simulink model "Simulation_CircularSensor"  (R2020a)
settings: Solver=VariableStepAuto  StartTime=0.0  StopTime=10  RelTol=1e-3
values from neighbouring files (symbols this model uses):
  L = 0    [CircularSensorTest.m]    (also in init.m = 0 * scale; polyTest.m = 10)
  Pixels = [0 0 0 0 0 0 0 0 0 0 0 0 ... (1000000 elements, 1000x1000)]    [CrossMap.mat]    (also in GenerateCourseData.m = zeros(Height, Width); Pixels.mat = [0 0 0 0 0 0 0 0 0 0 0 0 ... (19600 elements, 140x140)])
  scale = 1    [GenerateCourseData.m]
  SensorAngle = 60    [CircularSensorTest.m]    (also in init.m)
  SensorNumber = 3    [CircularSensorTest.m]    (also in animation2.m = evalin('base', 'SensorNumber'); init.m)
  SensorRadius = 40    [CircularSensorTest.m]    (also in init.m = 50 * scale)
  SensorRange = 20    [CircularSensorTest.m]    (also in animation2.m = evalin('base', 'SensorRange'); init.m = 25 * scale)
  Tvelo = 0.1    [init.m]
undefined symbols (not defined in the file or in its folder): DiscIntNeverNeededParam
settings Model: SimulationMode=rapid-accelerator  Creator=robot  LastModifiedBy=under

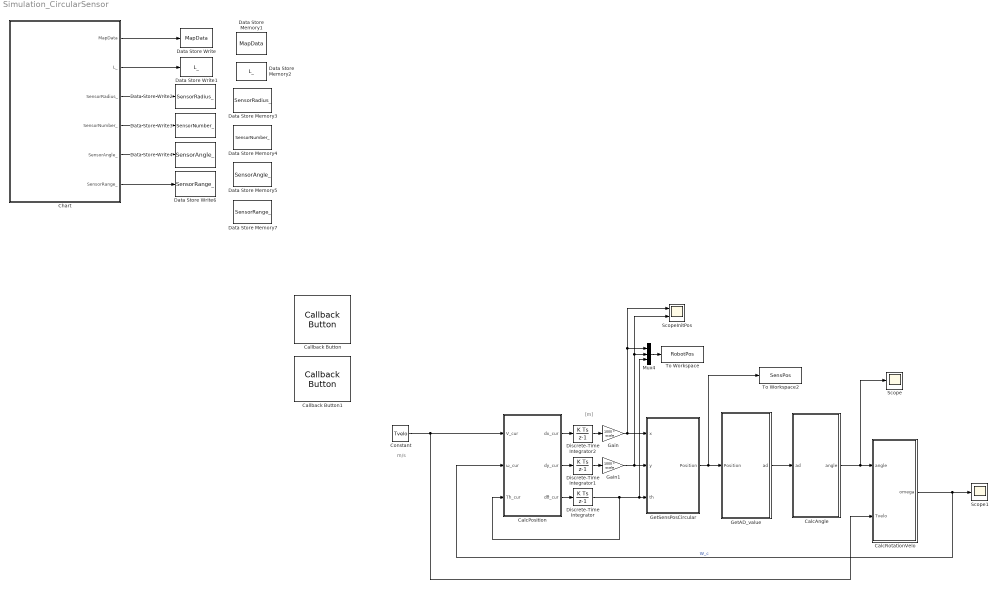
== system Simulation_CircularSensor ==
  note: [m]
  note: m/s
  CalcAngle : MATLAB Function  TreatAsAtomicUnit=on
  CalcPosition : Subsystem
  CalcRotationVelo : MATLAB Function  TreatAsAtomicUnit=on
  Callback Button : CallbackButton  ButtonText=Generata Course Data
      settings: ClickFcn=run('GenerateCourseData.m')
  Callback Button1 : CallbackButton  ButtonText=Initialize
      settings: ClickFcn=run('init.m')
  Chart : Stateflow chart  TreatAsAtomicUnit=on
  Constant : Constant  Value=Tvelo
  Data Store Memory1 : DataStoreMemory  DataStoreName=MapData  ReadBeforeWriteMsg=warning  WriteAfterWriteMsg=warning  WriteAfterReadMsg=warning  VectorParams1D=off  ShowAdditionalParam=off  OutDataTypeStr=double  Dimensions=[1000 ; 1000]
  Data Store Memory2 : DataStoreMemory  DataStoreName=L_  ReadBeforeWriteMsg=warning  WriteAfterWriteMsg=warning  WriteAfterReadMsg=warning  VectorParams1D=off  ShowAdditionalParam=off  OutDataTypeStr=double  Dimensions=1
  Data Store Memory3 : DataStoreMemory  DataStoreName=SensorRadius_  ReadBeforeWriteMsg=warning  WriteAfterWriteMsg=warning  WriteAfterReadMsg=warning  VectorParams1D=off  ShowAdditionalParam=off  OutDataTypeStr=double  Dimensions=1
  Data Store Memory4 : DataStoreMemory  DataStoreName=SensorNumber_  ReadBeforeWriteMsg=warning  WriteAfterWriteMsg=warning  WriteAfterReadMsg=warning  VectorParams1D=off  ShowAdditionalParam=off  OutDataTypeStr=double  Dimensions=1
  Data Store Memory5 : DataStoreMemory  DataStoreName=SensorAngle_  ReadBeforeWriteMsg=warning  WriteAfterWriteMsg=warning  WriteAfterReadMsg=warning  VectorParams1D=off  ShowAdditionalParam=off  OutDataTypeStr=double  Dimensions=1
  Data Store Memory7 : DataStoreMemory  DataStoreName=SensorRange_  ReadBeforeWriteMsg=warning  WriteAfterWriteMsg=warning  WriteAfterReadMsg=warning  VectorParams1D=off  ShowAdditionalParam=off  OutDataTypeStr=double  Dimensions=1
  Data Store Write : DataStoreWrite  DataStoreName=MapData
  Data Store Write1 : DataStoreWrite  DataStoreName=L_
  Data Store Write2 : DataStoreWrite  DataStoreName=SensorRadius_
  Data Store Write3 : DataStoreWrite  DataStoreName=SensorNumber_
  Data Store Write4 : DataStoreWrite  DataStoreName=SensorAngle_
  Data Store Write6 : DataStoreWrite  DataStoreName=SensorRange_
  Discrete-Time Integrator : DiscreteIntegrator  SampleTime=-1  ICPrevOutput=DiscIntNeverNeededParam  ICPrevScaledInput=DiscIntNeverNeededParam
  Discrete-Time Integrator1 : DiscreteIntegrator  InitialCondition=0.15  SampleTime=-1  ICPrevOutput=DiscIntNeverNeededParam  ICPrevScaledInput=DiscIntNeverNeededParam
  Discrete-Time Integrator2 : DiscreteIntegrator  InitialCondition=0.5  SampleTime=-1  ICPrevOutput=DiscIntNeverNeededParam  ICPrevScaledInput=DiscIntNeverNeededParam
  Gain : Gain  Gain=1000 * scale
  Gain1 : Gain  Gain=1000 * scale
  GetAD_value : MATLAB Function  TreatAsAtomicUnit=on
  GetSensPosCircular : MATLAB Function  TreatAsAtomicUnit=on
  Mux4 : Mux  Inputs=3
  Scope : Scope
  Scope1 : Scope
  ScopeInitPos : Scope  NumInputPorts=2
  To Workspace : ToWorkspace  VariableName=RobotPos  SampleTime=-1
  To Workspace2 : ToWorkspace  VariableName=SensPos  SaveFormat=Structure  SampleTime=-1
  wires:
  Constant/1 -> CalcPosition/1(V_cur), CalcRotationVelo/2(Tvelo)
  CalcPosition/3(dθ_cur) -> Discrete-Time Integrator/1
  Discrete-Time Integrator/1 -> CalcPosition/3(Th_cur), Mux4/3, GetSensPosCircular/3(th)
  Mux4/1 -> To Workspace/1
  GetSensPosCircular/1(Position) -> To Workspace2/1, GetAD_value/1(Position)
  Discrete-Time Integrator2/1 -> Gain/1
  Discrete-Time Integrator1/1 -> Gain1/1
  CalcPosition/1(dx_cur) -> Discrete-Time Integrator2/1
  CalcPosition/2(dy_cur) -> Discrete-Time Integrator1/1
  Gain/1 -> ScopeInitPos/1, Mux4/1, GetSensPosCircular/1(x)
  Gain1/1 -> ScopeInitPos/2, Mux4/2, GetSensPosCircular/2(y)
  Chart/1(MapData) -> Data Store Write/1
  Chart/2(L_) -> Data Store Write1/1
  Chart/3(SensorRadius_) -> Data Store Write2/1
  Chart/4(SensorNumber_) -> Data Store Write3/1
  Chart/5(SensorAngle_) -> Data Store Write4/1
  Chart/6(SensorRange_) -> Data Store Write6/1
  GetAD_value/1(ad) -> CalcAngle/1(ad)
  CalcAngle/1(angle) -> Scope/1, CalcRotationVelo/1(angle)
  CalcRotationVelo/1(omega) -> CalcPosition/2(ω_cur), Scope1/1  "W_c"

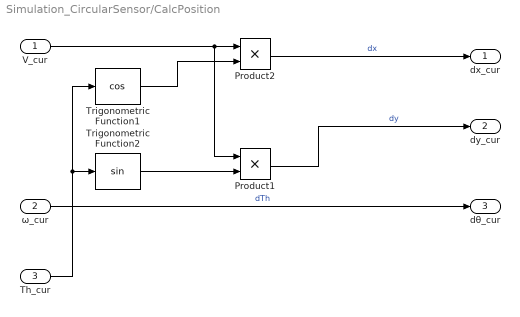
== system Simulation_CircularSensor/CalcPosition ==
  V_cur : Inport
  ω_cur : Inport  Port=2
  Th_cur : Inport  Port=3
  Product1 : Product
  Product2 : Product
  Trigonometric Function1 : Trigonometry  Operator=cos
  Trigonometric Function2 : Trigonometry
  dx_cur : Outport  VectorParamsAs1DForOutWhenUnconnected=off
  dy_cur : Outport  Port=2  VectorParamsAs1DForOutWhenUnconnected=off
  dθ_cur : Outport  Port=3  VectorParamsAs1DForOutWhenUnconnected=off
  wires:
  V_cur/1 -> Product2/1, Product1/1
  Trigonometric Function1/1 -> Product2/2
  Th_cur/1 -> Trigonometric Function2/1, Trigonometric Function1/1
  Product2/1 -> dx_cur/1  "dx"
  Product1/1 -> dy_cur/1  "dy"
  Trigonometric Function2/1 -> Product1/2
  ω_cur/1 -> dθ_cur/1  "dTh"

== matlab function Simulation_CircularSensor/CalcAngle ==
  data: ad input size=[1. 20]; angle output; SensorAngle_ data_store_memory; SensorNumber_ data_store_memory
function angle = fcn(ad)

    global SensorAngle_;
    global SensorNumber_
    
    AngleBetweenSensor = deg2rad(SensorAngle_ / SensorNumber_); %[rad]
    AllSensorNumer = SensorNumber_ * 2 + 1;
    CenterNumber = ceil(AllSensorNumer / 2); %Number of center sensor

    [~, Index] = max(ad);
    
    if Index == 1
        NormAD = [0, ad(1, Index) / ad(1, Index), ad(1, Index + 1) / ad(1, Index)];
    elseif Index == AllSensorNumer
        NormAD = [ad(1, Index - 1) / ad(1, Index), ad(1, Index) / ad(1, Index), 0];
    else
        NormAD = [ad(1, Index - 1) / ad(1, Index), ad(1, Index) / ad(1, Index), ad(1, Index + 1) / ad(1, Index)];
    end
    
    ratio = NormAD(1) -  NormAD(3);
    StandardAngle = (CenterNumber - Index(1, 1)) * AngleBetweenSensor;
    DeltaTheta = (AngleBetweenSensor / 2)  * ratio;
    
    
    angle = StandardAngle + DeltaTheta;

end

== matlab function Simulation_CircularSensor/GetSensPosCircular ==
  data: x input; y input; th input; Position output size=[2, 20]; L_ data_store_memory; SensorNumber_ data_store_memory; SensorAngle_ data_store_memory; SensorRadius_ data_store_memory
function Position = fcn(x, y, th)
global L_;
global SensorNumber_;
global SensorAngle_;
global SensorRadius_;

Origin = [x + L_ * cos(th); y + L_ * sin(th)];

AngleBetweenSensor = deg2rad(SensorAngle_ / SensorNumber_); %[rad]
AllSensorNumer = SensorNumber_ * 2 + 1;
InitialSensPos = zeros(2, AllSensorNumer); %Initialization
CenterNumber = ceil(AllSensorNumer / 2); %Number of center sensor
InitialSensPos(:, CenterNumber) = Origin + [SensorRadius_; 0]; % Position of center sensor

DeltaTh = 0;
for i = 1 : SensorNumber_ 
    DeltaTh = DeltaTh + AngleBetweenSensor;
    InitialSensPos(:, CenterNumber + i) = [cos(DeltaTh), -sin(DeltaTh) ; sin(DeltaTh), cos(DeltaTh)] * (InitialSensPos(:, CenterNumber) - Origin) + Origin;
    InitialSensPos(1, CenterNumber - i) = InitialSensPos(1, CenterNumber + i);
    InitialSensPos(2, CenterNumber - i) = InitialSensPos(2, CenterNumber) - (InitialSensPos(2, CenterNumber+ i) - InitialSensPos(2, CenterNumber)); 
end

RotatedSensPos = zeros(2, AllSensorNumer);
for i = 1 : AllSensorNumer
    RotatedSensPos(:, i) = [cos(th), -sin(th) ; sin(th), cos(th)] * (InitialSensPos(:, i) - Origin) + Origin;
end
    
Position = RotatedSensPos;

== matlab function Simulation_CircularSensor/CalcRotationVelo ==
  settings: updateMethod=DISCRETE
  data: angle input; omega output; L_ data_store_memory; Tvelo input
function omega = fcn(angle, Tvelo)
    global L_
    
    if angle ~= 0
        Radius = L_ / tan(angle);
    else
        Radius = 9e10;
        
    end
    
    omega = -Tvelo / (Radius * 1e-3);    
end

== matlab function Simulation_CircularSensor/GetAD_value ==
  settings: updateMethod=DISCRETE
  data: Position input size=[2. 20]; ad output size=[1, 20]; MapData data_store_memory; SensorRange_ data_store_memory; SensorNumber_ data_store_memory; SensorRadius_ data_store_memory
function ad = fcn(Position)
global SensorRadius_;
global SensorNumber_;
global MapData;

Trimming = zeros(SensorRadius_, SensorRadius_);
AllSensorNumer = SensorNumber_ * 2 + 1;
ad = zeros(1, AllSensorNumer);
xMax = numel(MapData(1, :));
yMax = numel(MapData(:, 1));

for k = 1 : AllSensorNumer
    x = Position(1, k);
    y = Position(2, k);
    for i = 1 : SensorRadius_
        for j = 1 : SensorRadius_  
            if (x - ceil(SensorRadius_ / 2) + j > 0) && (x + ceil(SensorRadius_ / 2) + j < xMax) && (y -ceil( SensorRadius_ / 2) + i > 0) && (y - ceil(SensorRadius_ / 2) + i < yMax)
                Trimming(i, j) = MapData(ceil((y - SensorRadius_ / 2) + i), ceil((x - SensorRadius_ / 2) + j));
            else
                Trimming(i, j) = NaN(1);
            end  
        end      
    end
    ad(k) = mean(Trimming, 'all');
end

% Trimming

% ad = 0;
end

== stateflow chart Simulation_CircularSensor/Chart ==
  state GetMap
    entry:
    MapData = Pixels;
    L_ = L;
    SensorRadius_ = SensorRadius;
    SensorNumber_ = SensorNumber;
    SensorAngle_ = SensorAngle;
    SensorRange_ = SensorRange;
    flag = 1;
  state Idle
  (default) -> GetMap
  GetMap -> Idle : [flag == 1]
  data: Pixels parameter; MapData output; L_ output; SensorRadius_ output; SensorNumber_ output; SensorAngle_ output; flag local; SensorRadius parameter; SensorAngle parameter; SensorNumber parameter; SensorRange parameter; SensorRange_ output; L parameter
